simulink model "BE2et5_simu"  (R2018b)
settings: Solver=VariableStepAuto  StartTime=0.0  StopTime=120  RelTol=1e-3
values from neighbouring files (symbols this model uses):
  A = [1.5 0 0 0; 0 3 0 0; 0 0 0.5 0; 0 0 0 0.9]    [BE1.m]    (also in BE2a5.m = [a 0 ; (3*alpha0*v0^2)/(J*w0) (-alpha0*v0^3)/(J*w0^2)])
  B = [1 2; 1 2; 0 0; 1 2]    [BE1.m]    (also in BE2a5.m = [0 ; -Ke/J])
  C = [1 1 1 0; 0 1 3 1]    [BE1.m]    (also in BE2a5.m = [0  1])
  F = inv(R + B'*P*B)*B'*P*A    [BE1.m]    (also in BE2a5.m = lqr(sysC, Q, R))
  K = lqr(A',C',W,V)'    [BE2a5.m]
  L = [-lambda/r 1]    [BE2a5.m]
  x0 = [2 2 2 2]'    [BE1.m]    (also in BE2a5.m = [v0, w0])
settings Model: Creator=piffercg  LastModifiedBy=piffercg

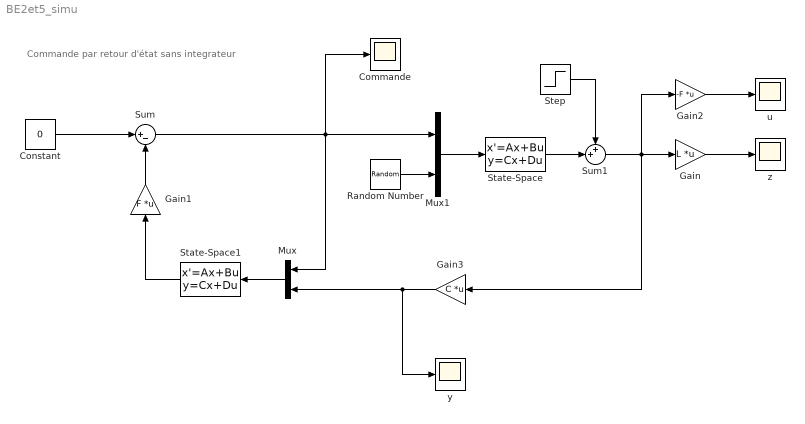
== system BE2et5_simu ==
  note: Commande par retour d'état sans integrateur
  Commande : Scope
  Constant : Constant  Value=0
  Gain : Gain  Gain=L  Multiplication=Matrix(K*u) (u vector)
  Gain1 : Gain  Gain=F  Multiplication=Matrix(K*u)
  Gain2 : Gain  Gain=-F  Multiplication=Matrix(K*u) (u vector)
  Gain3 : Gain  Gain=C  Multiplication=Matrix(K*u) (u vector)
  Mux : Mux  Inputs=2
  Mux1 : Mux  Inputs=2
  Random Number : RandomNumber  SampleTime=1
  State-Space : StateSpace  A=A  B=[B E]  C=eye(2)  D=[0 0; 0 0]  InitialCondition=x0
  State-Space1 : StateSpace  A=A-K*C  B=[B E]  C=eye(2)  D=[0 0; 0 0]  InitialCondition=0
  Step : Step  Time=100  After=0  SampleTime=0
  Sum : Sum  Inputs=|+-
  Sum1 : Sum  Inputs=++|
  u : Scope
  y : Scope
  z : Scope
  wires:
  Random Number/1 -> Mux1/2
  Sum/1 -> Commande/1, Mux/1, Mux1/1
  Mux1/1 -> State-Space/1
  State-Space/1 -> Sum1/2
  Step/1 -> Sum1/1
  Sum1/1 -> Gain3/1, Gain2/1, Gain/1
  Mux/1 -> State-Space1/1
  Gain1/1 -> Sum/2
  State-Space1/1 -> Gain1/1
  Constant/1 -> Sum/1
  Gain/1 -> z/1
  Gain2/1 -> u/1
  Gain3/1 -> y/1, Mux/2
